simulink model "leo_chukwuezi_sim_3pt4_sipro"  (R2024b)
settings: Solver=VariableStepAuto  StartTime=0.0  StopTime=8.0  MaxStep=1e-4  RelTol=1e-3
values from neighbouring files (symbols this model uses):
  G = 1    [leo_chukwuezi_sipro_lab2.m]
  wo = 2    [leo_chukwuezi_sipro_lab2.m]
undefined symbols (not defined in the file or in its folder): dend, dspblkCoreblockFVToolHelper, gcbh, numd
settings Model: Creator=DELL E7320  LastModifiedBy=DELL E7320

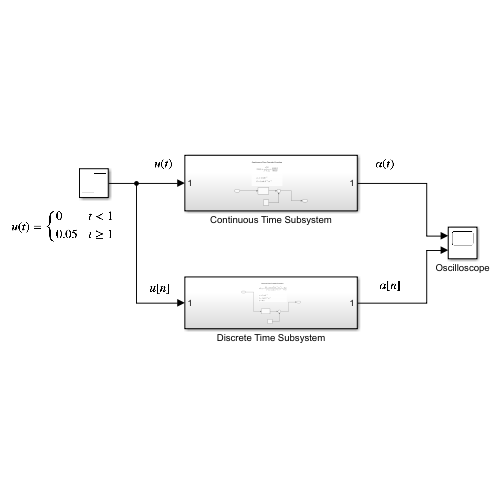
[thumbnail: Simulink's stored preview of the top-level diagram]
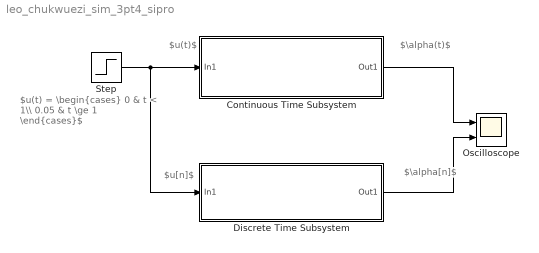
== system leo_chukwuezi_sim_3pt4_sipro ==
  note: $\alpha(t)$
  note: $u(t)$
  note: $u[n]$
  note: $\alpha[n]$
  note: $u(t) = \begin{cases} 0 & t < 1\\ 0.05 & t \ge 1 \end{cases}$
  Continuous Time Subsystem : Subsystem
  Discrete Time Subsystem : Subsystem
  Oscilloscope : Scope  NumInputPorts=2
  Step : Step  After=0.05  SampleTime=0.1
  wires:
  Step/1 -> Discrete Time Subsystem/1(In1), Continuous Time Subsystem/1(In1)
  Continuous Time Subsystem/1(Out1) -> Oscilloscope/1
  Discrete Time Subsystem/1(Out1) -> Oscilloscope/2

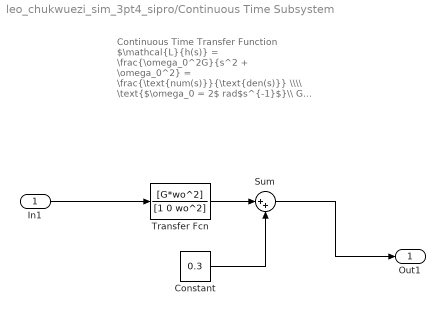
== system leo_chukwuezi_sim_3pt4_sipro/Continuous Time Subsystem ==
  note: Continuous Time Transfer Function
      |
      | $\mathcal{L}{h(s)} = \frac{\omega_0^2G}{s^2 + \omega_0^2} = \frac{\text{num(s)}}{\text{den(s)}} \\\\ \text{$\omega_0 = 2$ rad$s^{-1}$}\\ G = 1\, \text{rad.}N^{-1}.m^{-1}\\ %Ts = 0.1\,s$
  In1 : Inport
  Constant : Constant  Value=0.3
  Sum : Sum  Inputs=|++
  Transfer Fcn : TransferFcn  Numerator=[G*wo^2]  Denominator=[1 0 wo^2]
  Out1 : Outport
  wires:
  Constant/1 -> Sum/2
  Transfer Fcn/1 -> Sum/1
  In1/1 -> Transfer Fcn/1
  Sum/1 -> Out1/1

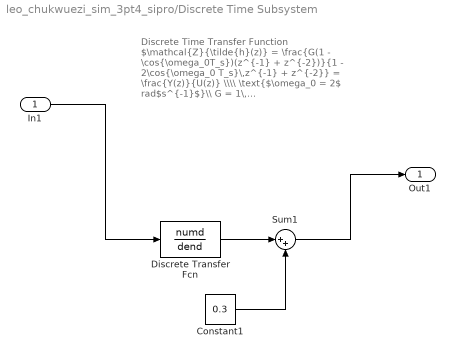
== system leo_chukwuezi_sim_3pt4_sipro/Discrete Time Subsystem ==
  note: Discrete Time Transfer Function
      |
      | $\mathcal{Z}{\tilde{h}(z)} = \frac{G(1 - \cos{\omega_0T_s})(z^{-1} + z^{-2})}{1 - 2\cos{\omega_0 T_s}\,z^{-1} + z^{-2}} = \frac{Y(z)}{U(z)} \\\\ \text{$\omega_0 = 2$ rad$s^{-1}$}\\ G = 1\, \text{rad.}N^{-1}.m^{-1}\\ T_s = 0.1\,s$
  In1 : Inport
  Constant1 : Constant  Value=0.3
  Discrete Transfer Fcn : DiscreteTransferFcn  LoadFcn=dspblkCoreblockFVToolHelper(gcbh,'load');  Numerator=numd  Denominator=dend
      settings: CopyFcn=dspblkCoreblockFVToolHelper(gcbh,'copy');  DeleteFcn=dspblkCoreblockFVToolHelper(gcbh,'close');  ModelCloseFcn=dspblkCoreblockFVToolHelper(gcbh,'close');  PreSaveFcn=dspblkCoreblockFVToolHelper(gcbh,'presave');  PostSaveFcn=dspblkCoreblockFVToolHelper(gcbh,'postsave');  CloseFcn=dspblkCoreblockFVToolHelper(gcbh,'close');
  Sum1 : Sum  Inputs=|++
  Out1 : Outport
  wires:
  Constant1/1 -> Sum1/2
  In1/1 -> Discrete Transfer Fcn/1
  Sum1/1 -> Out1/1
  Discrete Transfer Fcn/1 -> Sum1/1
